simulink library "Motor_Power_v2"  (R2020b)
settings: Solver=VariableStepAuto  StartTime=0.0  StopTime=10.0  RelTol=1e-3
values from neighbouring files (symbols this model uses):
  motor_power = motor_data(2:12,2:end)    [init.m]
  motor_speed = motor_data(2:12,1)    [init.m]
  motor_torque = motor_data(1,2:end)    [init.m]
  P_consumer = 1050    [init.m]
settings Model: Creator=janbantle  LastModifiedBy=Johnathy

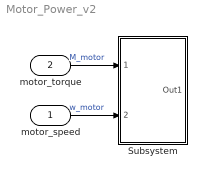
== system Motor_Power_v2 ==
  motor_speed : Inport
  motor_torque : Inport  Port=2
  Subsystem : Subsystem
  wires:
  motor_torque/1 -> Subsystem/1(motor_torque)  "M_motor"
  motor_speed/1 -> Subsystem/2(motor_speed)  "w_motor"

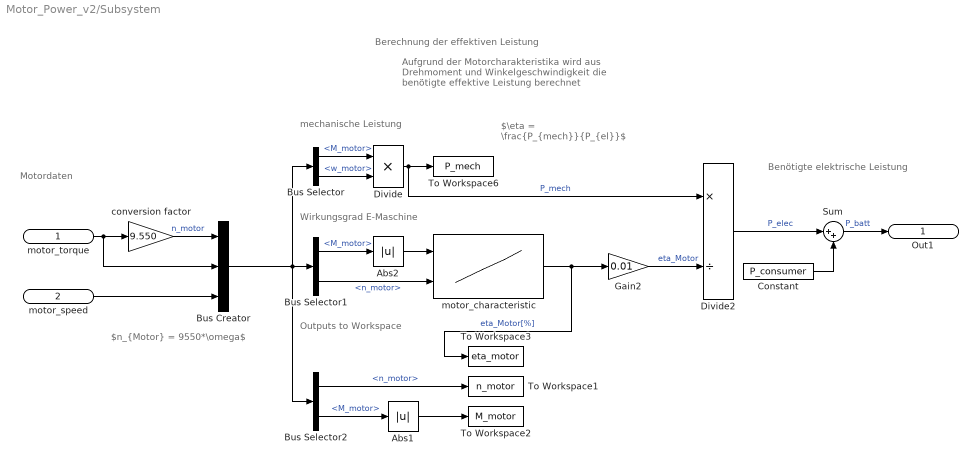
== system Motor_Power_v2/Subsystem ==
  note: $\eta = \frac{P_{mech}}{P_{el}}$
  note: Benötigte elektrische Leistung
  note: Wirkungsgrad E-Maschine
  note: mechanische Leistung
  note: Motordaten
  note: Aufgrund der Motorcharakteristika wird
      | aus Drehmoment und Winkelgeschwindigkeit
      | die benötigte effektive Leistung berechnet
  note: Berechnung der effektiven Leistung
  note: $n_{Motor} = 9550*\omega$
  note: Outputs to Workspace
  motor_torque : Inport
  motor_speed : Inport  Port=2
  Abs1 : Abs
  Abs2 : Abs
  Bus Creator : BusCreator  Inputs=3
  Bus Selector : BusSelector  OutputSignals=M_motor,w_motor
  Bus Selector1 : BusSelector  OutputSignals=M_motor,n_motor
  Bus Selector2 : BusSelector  OutputSignals=n_motor,M_motor
  Constant : Constant  Value=P_consumer
  Divide : Product  Inputs=**
  Divide2 : Product  Inputs=*/
  Gain2 : Gain  Gain=0.01
  Sum : Sum  Inputs=|++
  To Workspace1 : ToWorkspace  VariableName=n_motor  SampleTime=-1
  To Workspace2 : ToWorkspace  VariableName=M_motor  SampleTime=-1
  To Workspace3 : ToWorkspace  VariableName=eta_motor  SampleTime=-1
  To Workspace6 : ToWorkspace  VariableName=P_mech  SampleTime=-1
  conversion factor : Gain  Gain=9.550
  motor_characteristic : Lookup_n-D  BreakpointsForDimension1=motor_speed  BreakpointsForDimension2=motor_torque  BreakpointsForDimension3=[5, 7]  IndexSearchMethod=Linear search  Table=motor_power  InternalRulePriority=Speed  RndMeth=Simplest  InputSameDT=on
      settings: InputPortMap=u0,u1
  Out1 : Outport
  wires:
  motor_speed/1 -> Bus Creator/3
  conversion factor/1 -> Bus Creator/1  "n_motor"
  Abs1/1 -> To Workspace2/1
  Bus Selector2/1 -> To Workspace1/1  "<n_motor>"
  Bus Selector2/2 -> Abs1/1  "<M_motor>"
  Bus Selector1/1 -> Abs2/1  "<M_motor>"
  Bus Selector/1 -> Divide/1  "<M_motor>"
  Bus Selector/2 -> Divide/2  "<w_motor>"
  motor_characteristic/1 -> To Workspace3/1, Gain2/1  "eta_Motor[%]"
  Abs2/1 -> motor_characteristic/1
  motor_torque/1 -> conversion factor/1, Bus Creator/2
  Divide/1 -> Divide2/1, To Workspace6/1  "P_mech"
  Gain2/1 -> Divide2/2  "eta_Motor"
  Divide2/1 -> Sum/1  "P_elec"
  Constant/1 -> Sum/2
  Bus Creator/1 -> Bus Selector1/1, Bus Selector2/1, Bus Selector/1
  Bus Selector1/2 -> motor_characteristic/2  "<n_motor>"
  Sum/1 -> Out1/1  "P_batt"
